simulink model "project_model"  (R2025a)
settings: Solver=FixedStepAuto  StartTime=0.0  StopTime=10.0  FixedStep=1e-3  RelTol=1e-3  EnableMultiTasking=on
undefined symbols (not defined in the file): D2, D5, PTA2, PTB9
libraries: frdmk64flib x3
settings Model: ExtModeTrigDuration=5  Creator=justi  LastModifiedBy=justi
settings OptimizationCC: DefaultParameterBehavior=Inlined  EnhancedBackFolding=on  PassReuseOutputArgsAs=Individual arguments  ZeroExternalMemoryAtStartup=off  ZeroInternalMemoryAtStartup=off  MaxStackSize=64  OptimizeBlockOrder=speed  DifferentSizesBufferReuse=on  OptimizationCustomize=off  EfficientTunableParamExpr=on
settings DebuggingCC: ParameterTunabilityLossMsg=error
settings HardwareCC: ProdBitPerPointer=32.0  ProdBitPerSizeT=32.0  ProdBitPerPtrDiffT=32.0  ProdLargestAtomicInteger=Long  ProdLargestAtomicFloat=Double  ProdWordSize=32.0  ProdHWDeviceType=ARM Compatible->ARM Cortex
settings SFSimCC: MATLABDynamicMemAlloc=off
settings RTWCC: SystemTargetFile=ert.tlc  HardwareBoard=NXP FRDM-K64F  TLCOptions="-aInlineSetEventsForThisBaseRateFcn=TLC_FALSE -aSuppressMultiTaskScheduler=TLC_FALSE  -aRateBasedStepFcn=0"  TemplateMakefile=ert_default_tmf  Toolchain=GNU Tools for ARM Embedded Processors  Description=Embedded Coder
settings CodeAppCC: ForceParamTrailComments=on  IgnoreCustomStorageClasses=off  OperatorAnnotations=on  SimulinkDataObjDesc=on  SFDataObjDesc=on  InsertBlockDesc=on
settings ERTTargetCC: ExtModeTransport=4.0  ExtModeStaticAlloc=off  ExtModeMexFile=sendToCommService  ExtModeIntrfLevel=Level1

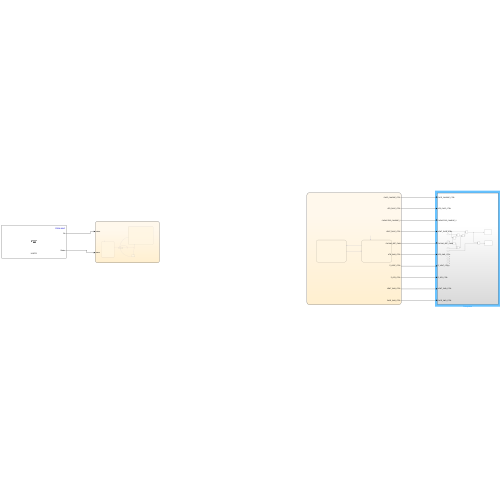
[thumbnail: Simulink's stored preview of the top-level diagram]
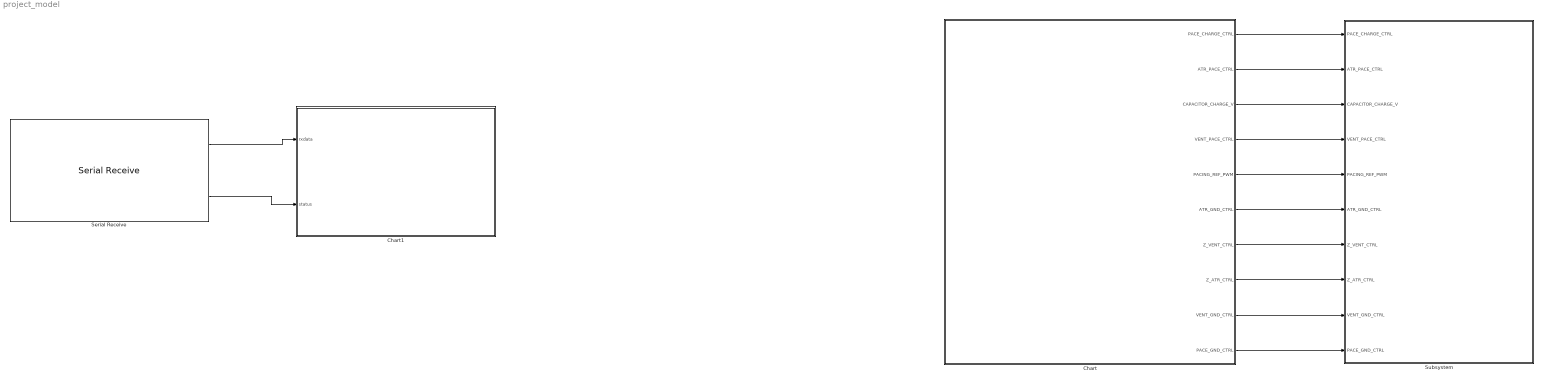
== system project_model ==
  Chart : Stateflow chart  TreatAsAtomicUnit=on
  Chart1 : Stateflow chart  TreatAsAtomicUnit=on
  Serial Receive : frdmk64flib/Serial Receive  SCIModule=0  Baudrate=uint32(9600)  Parity=None  StopBits=1  HardwareFlowControl=None  ByteOrder=LittleEndian  DataType=uint8  DataLength=10  BlockingMode=off  OutputStatus=on  SampleTime=0.1
  Subsystem : Subsystem
  wires:
  Serial Receive/1 -> Chart1/1(rxdata)
  Serial Receive/2 -> Chart1/2(status)
  Chart/1(PACE_CHARGE_CTRL) -> Subsystem/1(PACE_CHARGE_CTRL)
  Chart/2(ATR_PACE_CTRL) -> Subsystem/2(ATR_PACE_CTRL)
  Chart/3(CAPACITOR_CHARGE_V) -> Subsystem/3(CAPACITOR_CHARGE_V)
  Chart/4(VENT_PACE_CTRL) -> Subsystem/4(VENT_PACE_CTRL)
  Chart/5(PACING_REF_PWM) -> Subsystem/5(PACING_REF_PWM)
  Chart/6(ATR_GND_CTRL) -> Subsystem/6(ATR_GND_CTRL)
  Chart/7(Z_VENT_CTRL) -> Subsystem/7(Z_VENT_CTRL)
  Chart/8(Z_ATR_CTRL) -> Subsystem/8(Z_ATR_CTRL)
  Chart/9(VENT_GND_CTRL) -> Subsystem/9(VENT_GND_CTRL)
  Chart/10(PACE_GND_CTRL) -> Subsystem/10(PACE_GND_CTRL)

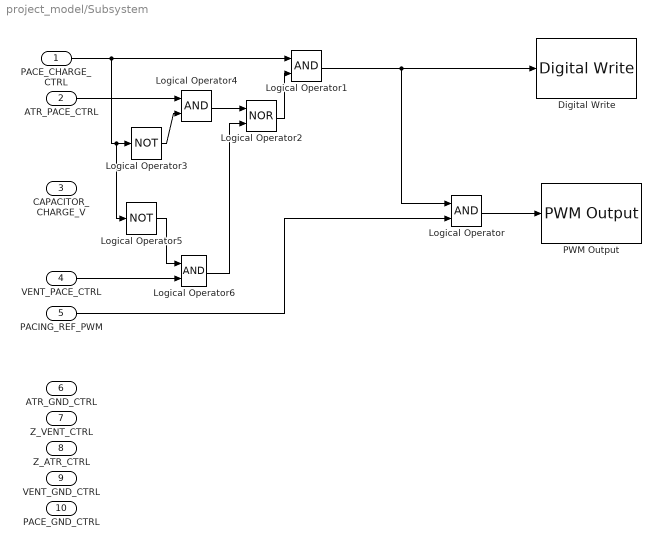
== system project_model/Subsystem ==
  PACE_CHARGE_CTRL : Inport
  ATR_PACE_CTRL : Inport  Port=2
  CAPACITOR_CHARGE_V : Inport  Port=3
  VENT_PACE_CTRL : Inport  Port=4
  PACING_REF_PWM : Inport  Port=5
  ATR_GND_CTRL : Inport  Port=6
  Z_VENT_CTRL : Inport  Port=7
  Z_ATR_CTRL : Inport  Port=8
  VENT_GND_CTRL : Inport  Port=9
  PACE_GND_CTRL : Inport  Port=10
  Digital Write : frdmk64flib/Digital Write  Whichpin=PTB9 (D2)
  Logical Operator{,1,4,6} (4 alike) : Logic  AllPortsSameDT=off  OutDataTypeStr=boolean
  Logical Operator2 : Logic  Operator=NOR  AllPortsSameDT=off  OutDataTypeStr=boolean
  Logical Operator3 : Logic  Operator=NOT  AllPortsSameDT=off  OutDataTypeStr=boolean
  Logical Operator5 : Logic  Operator=NOT  AllPortsSameDT=off  OutDataTypeStr=boolean
  PWM Output : frdmk64flib/PWM Output  Whichpin=PTA2 (D5)  InitialFrequency=2000  InitialDutyCycle=0
  wires:
  Logical Operator/1 -> PWM Output/1
  Logical Operator1/1 -> Logical Operator/1, Digital Write/1
  Logical Operator2/1 -> Logical Operator1/2
  Logical Operator3/1 -> Logical Operator4/2
  ATR_PACE_CTRL/1 -> Logical Operator4/1
  Logical Operator4/1 -> Logical Operator2/1
  PACING_REF_PWM/1 -> Logical Operator/2
  PACE_CHARGE_CTRL/1 -> Logical Operator5/1, Logical Operator3/1, Logical Operator1/1
  VENT_PACE_CTRL/1 -> Logical Operator6/2
  Logical Operator5/1 -> Logical Operator6/1
  Logical Operator6/1 -> Logical Operator2/2

== stateflow chart project_model/Chart1 ==
  state SET_PARAM_
    entry:
    LOWER_RATE_LIMIT=typecast(rxdata(3:4),'uint16');
    UPPER_RATE_LIMIT=typecast(rxdata(5:6),'uint16');
    MAXIMUM_SENSOR_RATE=typecast(rxdata(7:8),'uint16');
    FIXED_AV_DELAY=typecast(rxdata(9:10),'uint16');
    DYNAMIC_AV_DELAY=typecast(rxdata(11:12),'uint16');
    SENSED_AV_DELAY_OFFSET=typecast(rxdata(13:14),'uint16');
    ATRIAL_AMPLITUDE=typecast(rxdata(15:16),'uint16');
    VENTRICULAR_AMPLITUDE=typecast(rxdata(17:18),'uint16');
    ATRIAL_PULSE_WIDTH=typecast(rxdata(19:20),'uint16');
    VENTRICULAR_PULSE_WIDTH=typecast(rxdata(21:22),'uint16');
    ATRIAL_SENSITIVITY=typecast(rxdata(23:24),'uint16');
    VENTRICULAR_SENSITIVITY=typecast(rxdata(25:26),'uint16');
    VRP=typecast(rxdata(27:28),'uint16');
    ARP=typecast(rxdata(29:30),'uint16');
    PVARP=typecast(rxdata(31:32),'uint16');
    PVARP_EXTENSION=typecast(rxdata(33:34),'uint16');
    HYSTERESIS=typecast(rxdata(35:36),'uint16');
    RATE_SMOOTHING=typecast(rxdata(37:38),'uint16');
    ATR_DURATION=typecast(rxdata(39:40),'uint16');
    ATR_FALLBACK_MODE=typecast(rxdata(41:42),'uint16');
    ATR_FALLBACK_TIME=typecast(rxdata(43:44),'uint16');
    ACTIVITY_THRESHOLD=typecast(rxdata(45:46),'uint16');
    REACTION_TIME=typecast(rxdata(47:48),'uint16');
    RESPONSE_FACTOR=typecast(rxdata(49:50),'uint16');
    RECOVERY_TIME=typecast(rxdata(51:52),'uint16');
  state INITIAL
    entry:
    LOWER_RATE_LIMIT = 0;
    UPPER_RATE_LIMIT = 0;
    MAXIMUM_SENSOR_RATE = 0;
    FIXED_AV_DELAY = 0;
    DYNAMIC_AV_DELAY = 0;
    SENSED_AV_DELAY_OFFSET = 0;
    ATRIAL_AMPLITUDE = 0;
    VENTRICULAR_AMPLITUDE = 0;
    ATRIAL_PULSE_WIDTH = 0;
    VENTRICULAR_PULSE_WIDTH = 0;
    ATRIAL_SENSITIVITY = 0;
    VENTRICULAR_SENSITIVITY = 0;
    VRP = 0; ARP = 0; PVARP = 0;
    PVARP_EXTENSION = 0;
    HYSTERESIS = 0;
    RATE_SMOOTHING = 0;
    ATR_DURATION = 0;
    ATR_FALLBACK_MODE = 0;
    ATR_FALLBACK_TIME = 0;
    ACTIVITY_THRESHOLD = 0;
    REACTION_TIME = 0;
    RESPONSE_FACTOR = 0;
    RECOVERY_TIME = 0;
  state STANDBY
    %Wait for COM
  state ECHO_PARAM
    entry:
    send_params();
  SET_PARAM_ -> STANDBY
  (default) -> INITIAL
  (junction 10) -> SET_PARAM_ [order 1] : [rx_data (2) == hex2dec('55')]
  (junction 8) -> STANDBY [order 2]
  INITIAL -> STANDBY
  STANDBY -> (junction 8) : [status == 0]
  (junction 8) -> (junction 10) [order 1] : [rx_data (1) == hex2dec('16')]
  (junction 10) -> ECHO_PARAM [order 2] : [rx_data (2) == hex2dec('22')]
  ECHO_PARAM -> STANDBY
  data: rxdata input; status input

== stateflow chart project_model/Chart ==
  state Discharge
    PACE_CHARGE_CTRL=0;
    PACE_GND_CTRL=1;
    ATR_PACE_CTRL=0;
    ATR_GND_CTRL=0;
    Z_ATR_CTRL=0;
    Z_VENT_CTRL=0;
    VENT_GND_CTRL=0;
    VENT_PACE_CTRL=0;
  state Charge
    ATR_PACE_CTRL=0;
    VENT_PACE_CTRL=0;
    PACING_REF_PWM=2000;%todo
    CAPACITOR_CHARGE_V=5;
    PACE_CHARGE_CTRL=1;
  (default) -> Charge
  Charge -> Discharge : [after(0.54,sec)]
  Discharge -> Charge : [after(0.54,sec)]
  data: PACE_CHARGE_CTRL output; ATR_PACE_CTRL output; CAPACITOR_CHARGE_V output; VENT_PACE_CTRL output; PACING_REF_PWM output; ATR_GND_CTRL output; Z_VENT_CTRL output; Z_ATR_CTRL output; VENT_GND_CTRL output; PACE_GND_CTRL output
